simulink subsystem "filter_1s2o"  (R2021b)
settings: Solver=VariableStepAuto  StartTime=0.0  StopTime=10.0  RelTol=1e-3
settings Model: Creator=torha  LastModifiedBy=torha

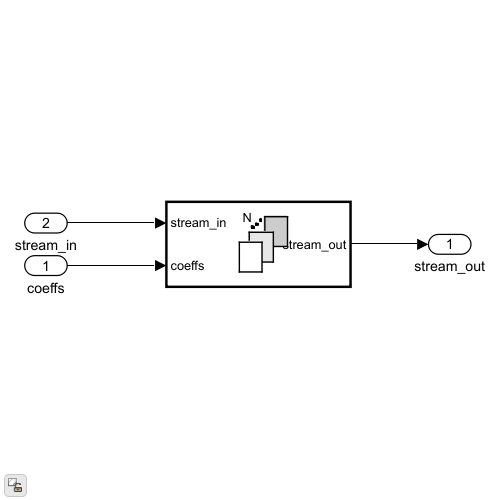
[thumbnail: Simulink's stored preview of the top-level diagram]
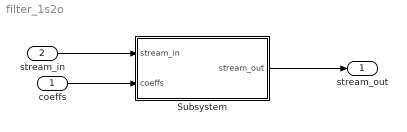
== system filter_1s2o ==
  coeffs : Inport
  stream_in : Inport  Port=2
  Subsystem : Subsystem
  stream_out : Outport
  wires:
  coeffs/1 -> Subsystem/2(coeffs)
  stream_in/1 -> Subsystem/1(stream_in)
  Subsystem/1(stream_out) -> stream_out/1

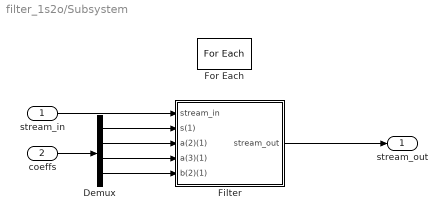
== system filter_1s2o/Subsystem ==
  stream_in : Inport  Partition=on  PartitionDimension=1  PartitionWidth=1  PartitionOffset=0
  coeffs : Inport  Port=2
  Demux : Demux
  Filter : Subsystem  Tag=FilterWizardSubSystem
      settings: ErrorFcn=dspFilterRealizedInBasicElemsAlgLoopErrFcnCallback
  For Each : ForEach  DisableCoverage=on
  stream_out : Outport  ConcatenationDimension=1
  wires:
  Demux/4 -> Filter/5(b(2)(1))
  Demux/3 -> Filter/4(a(3)(1))
  Demux/2 -> Filter/3(a(2)(1))
  Demux/1 -> Filter/2(s(1))
  stream_in/1 -> Filter/1(stream_in)
  coeffs/1 -> Demux/1
  Filter/1(stream_out) -> stream_out/1

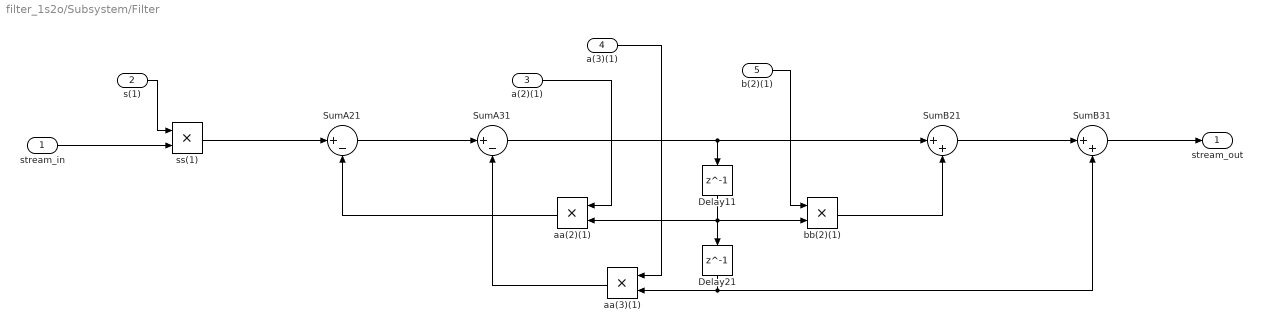
== system filter_1s2o/Subsystem/Filter ==
  stream_in : Inport
  s(1) : Inport  Port=2
  a(2)(1) : Inport  Port=3
  a(3)(1) : Inport  Port=4
  b(2)(1) : Inport  Port=5
  Delay11 : Delay  DelayLength=1  InitialCondition=0
  Delay21 : Delay  DelayLength=1  InitialCondition=0
  SumA21 : Sum  Inputs=|+-  RndMeth=Nearest  SaturateOnIntegerOverflow=on  OutDataTypeStr=Inherit: Same as first input
  SumA31 : Sum  Inputs=|+-  RndMeth=Nearest  SaturateOnIntegerOverflow=on  OutDataTypeStr=Inherit: Same as first input
  SumB21 : Sum  Inputs=|++  RndMeth=Nearest  SaturateOnIntegerOverflow=on  OutDataTypeStr=Inherit: Same as first input
  SumB31 : Sum  Inputs=|++  RndMeth=Nearest  SaturateOnIntegerOverflow=on  OutDataTypeStr=Inherit: Same as first input
  aa(2)(1) : Product
  aa(3)(1) : Product
  bb(2)(1) : Product
  ss(1) : Product
  stream_out : Outport
  wires:
  b(2)(1)/1 -> bb(2)(1)/1
  a(3)(1)/1 -> aa(3)(1)/1
  a(2)(1)/1 -> aa(2)(1)/1
  s(1)/1 -> ss(1)/1
  Delay21/1 -> SumB31/2, aa(3)(1)/2
  aa(3)(1)/1 -> SumA31/2
  bb(2)(1)/1 -> SumB21/2
  Delay11/1 -> aa(2)(1)/2, Delay21/1, bb(2)(1)/2
  aa(2)(1)/1 -> SumA21/2
  SumB31/1 -> stream_out/1
  SumB21/1 -> SumB31/1
  SumA31/1 -> Delay11/1, SumB21/1
  SumA21/1 -> SumA31/1
  ss(1)/1 -> SumA21/1
  stream_in/1 -> ss(1)/2
